simulink library "halout"  (R2021b)
settings: Solver=VariableStepAuto  StartTime=0.0  StopTime=10.0  RelTol=1e-3
undefined symbols (not defined in the file): C_TASK_5MS_S, FALSE, KHAL_CAN1FD1APS3E2E_flg, KHAL_CAN1FD1APS3TxReq_flg, KHAL_CAN1FD1VCU2E2E_flg, KHAL_CAN1FD1VCU2TxReq_flg, KHAL_CAN1FD1VCU3E2E_flg, KHAL_CAN1FD1VCU3TxReq_flg, KHAL_CAN1TxReq_flg, KHAL_CAN1VMCFCM1E2E_flg, KHAL_CAN1VMCFCM1TxReq_flg, KHAL_CAN2TxReq_flg, KHAL_CAN3FD3VCU1toNIDECTxReq_flg, KHAL_CAN3FD3VCU1TxReq_flg, KHAL_CAN3FD3VCU2E2E_flg, KHAL_CAN3FD3VCU2toNIDECE2E_flg, KHAL_CAN3FD3VCU2toNIDECTxReq_flg, KHAL_CAN3FD3VCU2TxReq_flg, KHAL_CAN3TxReq_flg, KHAL_CAN4FD4CE1000E2E_flg, KHAL_CAN4FD4CE1000TxReq_flg, KHAL_CAN4TxReq_flg, KHAL_CAN5TxReq_flg, KHAL_CAN6FD6APS3E2E_flg, KHAL_CAN6FD6APS3TxReq_flg, KHAL_CAN6FD6VCU2E2E_flg, KHAL_CAN6FD6VCU2TxReq_flg, KHAL_CAN6TxReq_flg, ONE_INT, TRUE, ZERO_INT
libraries: FVT_lib x549, simulink x244
(part 16 of 27)

== system halout/HAL_OUT/CAN1/FD1_VCU2_0x154/Byte_3 ==
  Fr_DriverTq : Inport
  BitwiseOR : simulink/Logic and Bit Operations/Bitwise Operator  logicop=OR  UseBitMask=off  BitMask=bin2dec('11011001')  BitMaskRealWorld=Stored Integer
  SignalPack : FVT_lib/hal/SignalPack  RightShiftCnt=0  BitMask=2^8-1  LeftShiftCnt=0
  UnitConverter : DataTypeConversion  OutDataTypeStr=uint8  RndMeth=Round
  UnitConverter1 : DataTypeConversion  OutDataTypeStr=uint16  RndMeth=Round
  convert_out : FVT_lib/hal/convert_out  gain=0.5  offset=-5300
  Byte_3 : Outport
  wires:
  BitwiseOR/1 -> Byte_3/1
  UnitConverter/1 -> BitwiseOR/1
  SignalPack/1 -> UnitConverter/1
  UnitConverter1/1 -> SignalPack/1
  convert_out/1 -> UnitConverter1/1
  Fr_DriverTq/1 -> convert_out/1

== system halout/HAL_OUT/CAN1/FD1_VCU2_0x154/Byte_4 ==
  Rr_DriverTq : Inport
  BitwiseOR : simulink/Logic and Bit Operations/Bitwise Operator  logicop=OR  UseBitMask=off  BitMask=bin2dec('11011001')  BitMaskRealWorld=Stored Integer
  SignalPack : FVT_lib/hal/SignalPack  RightShiftCnt=8  BitMask=2^8-1  LeftShiftCnt=0
  UnitConverter : DataTypeConversion  OutDataTypeStr=uint8  RndMeth=Round
  UnitConverter1 : DataTypeConversion  OutDataTypeStr=uint16  RndMeth=Round
  convert_out : FVT_lib/hal/convert_out  gain=0.5  offset=-5300
  Byte_4 : Outport
  wires:
  BitwiseOR/1 -> Byte_4/1
  UnitConverter/1 -> BitwiseOR/1
  SignalPack/1 -> UnitConverter/1
  UnitConverter1/1 -> SignalPack/1
  convert_out/1 -> UnitConverter1/1
  Rr_DriverTq/1 -> convert_out/1

== system halout/HAL_OUT/CAN1/FD1_VCU2_0x154/Byte_5 ==
  Rr_DriverTq : Inport
  BitwiseOR : simulink/Logic and Bit Operations/Bitwise Operator  logicop=OR  UseBitMask=off  BitMask=bin2dec('11011001')  BitMaskRealWorld=Stored Integer
  SignalPack : FVT_lib/hal/SignalPack  RightShiftCnt=0  BitMask=2^8-1  LeftShiftCnt=0
  UnitConverter : DataTypeConversion  OutDataTypeStr=uint8  RndMeth=Round
  UnitConverter1 : DataTypeConversion  OutDataTypeStr=uint16  RndMeth=Round
  convert_out : FVT_lib/hal/convert_out  gain=0.5  offset=-5300
  Byte_5 : Outport
  wires:
  BitwiseOR/1 -> Byte_5/1
  UnitConverter/1 -> BitwiseOR/1
  SignalPack/1 -> UnitConverter/1
  UnitConverter1/1 -> SignalPack/1
  convert_out/1 -> UnitConverter1/1
  Rr_DriverTq/1 -> convert_out/1

== system halout/HAL_OUT/CAN1/FD1_VCU2_0x154/Byte_6 ==
  ACC_CtrlAvail : Inport
  AccPedal_Override : Inport  Port=2
  BitwiseOR : simulink/Logic and Bit Operations/Bitwise Operator  logicop=OR  UseBitMask=off  NumInputPorts=2  BitMask=bin2dec('11011001')  BitMaskRealWorld=Stored Integer
  SignalPack : FVT_lib/hal/SignalPack  RightShiftCnt=0  BitMask=2^1-1  LeftShiftCnt=7
  SignalPack1 : FVT_lib/hal/SignalPack  RightShiftCnt=0  BitMask=2^1-1  LeftShiftCnt=6
  UnitConverter{,1..3} (4 alike) : DataTypeConversion  OutDataTypeStr=uint8  RndMeth=Round
  Byte_6 : Outport
  wires:
  BitwiseOR/1 -> Byte_6/1
  UnitConverter/1 -> BitwiseOR/1
  SignalPack/1 -> UnitConverter/1
  UnitConverter1/1 -> SignalPack/1
  ACC_CtrlAvail/1 -> UnitConverter1/1
  UnitConverter2/1 -> BitwiseOR/2
  SignalPack1/1 -> UnitConverter2/1
  UnitConverter3/1 -> SignalPack1/1
  AccPedal_Override/1 -> UnitConverter3/1

== system halout/HAL_OUT/CAN1/FD1_VCU2_0x154/CRC8_IfAction_Tx ==
  CAN_E2E_flg : Inport
  DataID1 : Inport  Port=2
  DataID2 : Inport  Port=3
  RawData : Inport  Port=4
  Data Type Conversion : DataTypeConversion  OutDataTypeStr=uint8
  If : If
  If Action Subsystem : Subsystem  TreatAsAtomicUnit=on
  If Action Subsystem1 : Subsystem  TreatAsAtomicUnit=on
  Merge : Merge
  CRC8 : Outport
  wires:
  If/2 -> If Action Subsystem/Action
  If/1 -> If Action Subsystem1/Action
  CAN_E2E_flg/1 -> [CAN_E2E_flg]
  DataID1/1 -> [DataID1]
  DataID2/1 -> [DataID2]
  RawData/1 -> [RawData]
  [CAN_E2E_flg] -> Data Type Conversion/1
  [DataID1] -> If Action Subsystem1/1(CAN_E2E_ID1)
  [DataID2] -> If Action Subsystem1/2(CAN_E2E_ID2)
  [RawData] -> If Action Subsystem1/3(Byte1)
  [RawData] -> If Action Subsystem/1(Byte1)
  If Action Subsystem1/1(CRC8_E2EResult) -> Merge/1
  If Action Subsystem/1(CRC8_Result) -> Merge/2
  Merge/1 -> CRC8/1
  Data Type Conversion/1 -> If/1

== system halout/HAL_OUT/CAN1/FD1_VCU2_0x154/CSVCU2CAN1 ==
  CSVCU2CAN1 : Inport
  Data Type Conversion : DataTypeConversion  OutDataTypeStr=uint8  RndMeth=Round
  CAN1_CS_VCU2_CAN1 : Outport
  wires:
  Data Type Conversion/1 -> CAN1_CS_VCU2_CAN1/1
  CSVCU2CAN1/1 -> Data Type Conversion/1

== system halout/HAL_OUT/CAN1/FD1_VCU2_0x154/DriverTq ==
  DriverTq : Inport
  Data Type Conversion : DataTypeConversion  OutDataTypeStr=uint16  RndMeth=Round
  convert_out : FVT_lib/hal/convert_out  gain=1  offset=-4300
  CAN1_DriverTq : Outport
  wires:
  Data Type Conversion/1 -> CAN1_DriverTq/1
  convert_out/1 -> Data Type Conversion/1
  DriverTq/1 -> convert_out/1

== system halout/HAL_OUT/CAN1/FD1_VCU2_0x154/FrDriverTq ==
  FrDriverTq : Inport
  Data Type Conversion : DataTypeConversion  OutDataTypeStr=uint16  RndMeth=Round
  convert_out : FVT_lib/hal/convert_out  gain=0.5  offset=-5300
  CAN1_Fr_DriverTq : Outport
  wires:
  Data Type Conversion/1 -> CAN1_Fr_DriverTq/1
  convert_out/1 -> Data Type Conversion/1
  FrDriverTq/1 -> convert_out/1

== system halout/HAL_OUT/CAN1/FD1_VCU2_0x154/RCVCU2CAN1 ==
  RCVCU2CAN1 : Inport
  Data Type Conversion : DataTypeConversion  OutDataTypeStr=uint8  RndMeth=Round
  CAN1_RC_VCU2_CAN1 : Outport
  wires:
  Data Type Conversion/1 -> CAN1_RC_VCU2_CAN1/1
  RCVCU2CAN1/1 -> Data Type Conversion/1

== system halout/HAL_OUT/CAN1/FD1_VCU2_0x154/RrDriverTq ==
  RrDriverTq : Inport
  Data Type Conversion : DataTypeConversion  OutDataTypeStr=uint16  RndMeth=Round
  convert_out : FVT_lib/hal/convert_out  gain=0.5  offset=-5300
  CAN1_Rr_DriverTq : Outport
  wires:
  Data Type Conversion/1 -> CAN1_Rr_DriverTq/1
  convert_out/1 -> Data Type Conversion/1
  RrDriverTq/1 -> convert_out/1

== system halout/HAL_OUT/CAN1/FD1_VCU2_0x154/VehActPwr ==
  VehActPwr : Inport
  Data Type Conversion : DataTypeConversion  OutDataTypeStr=uint32  RndMeth=Round
  convert_out : FVT_lib/hal/convert_out  gain=1  offset=-600000
  CAN1_VehActPwr : Outport
  wires:
  Data Type Conversion/1 -> CAN1_VehActPwr/1
  convert_out/1 -> Data Type Conversion/1
  VehActPwr/1 -> convert_out/1

== system halout/HAL_OUT/CAN1/FD1_VCU3_0x159/Byte_0 ==
  CS_VCU3_CAN1 : Inport
  BitwiseOR : simulink/Logic and Bit Operations/Bitwise Operator  logicop=OR  UseBitMask=off  BitMask=bin2dec('11011001')  BitMaskRealWorld=Stored Integer
  SignalPack : FVT_lib/hal/SignalPack  RightShiftCnt=0  BitMask=2^8-1  LeftShiftCnt=0
  UnitConverter : DataTypeConversion  OutDataTypeStr=uint8  RndMeth=Round
  UnitConverter1 : DataTypeConversion  OutDataTypeStr=uint8  RndMeth=Round
  Byte_0 : Outport
  wires:
  BitwiseOR/1 -> Byte_0/1
  UnitConverter/1 -> BitwiseOR/1
  SignalPack/1 -> UnitConverter/1
  UnitConverter1/1 -> SignalPack/1
  CS_VCU3_CAN1/1 -> UnitConverter1/1

== system halout/HAL_OUT/CAN1/FD1_VCU3_0x159/Byte_1 ==
  RC_VCU3_CAN1 : Inport
  BitwiseOR : simulink/Logic and Bit Operations/Bitwise Operator  logicop=OR  UseBitMask=off  BitMask=bin2dec('11011001')  BitMaskRealWorld=Stored Integer
  SignalPack : FVT_lib/hal/SignalPack  RightShiftCnt=0  BitMask=2^4-1  LeftShiftCnt=0
  UnitConverter : DataTypeConversion  OutDataTypeStr=uint8  RndMeth=Round
  UnitConverter1 : DataTypeConversion  OutDataTypeStr=uint8  RndMeth=Round
  Byte_1 : Outport
  wires:
  BitwiseOR/1 -> Byte_1/1
  UnitConverter/1 -> BitwiseOR/1
  SignalPack/1 -> UnitConverter/1
  UnitConverter1/1 -> SignalPack/1
  RC_VCU3_CAN1/1 -> UnitConverter1/1

== system halout/HAL_OUT/CAN1/FD1_VCU3_0x159/Byte_10 ==
  Rr_EDURealDrvOrBRgnTq : Inport
  BitwiseOR : simulink/Logic and Bit Operations/Bitwise Operator  logicop=OR  UseBitMask=off  BitMask=bin2dec('11011001')  BitMaskRealWorld=Stored Integer
  SignalPack : FVT_lib/hal/SignalPack  RightShiftCnt=8  BitMask=2^8-1  LeftShiftCnt=0
  UnitConverter : DataTypeConversion  OutDataTypeStr=uint8  RndMeth=Round
  UnitConverter1 : DataTypeConversion  OutDataTypeStr=uint16  RndMeth=Round
  convert_out : FVT_lib/hal/convert_out  gain=0.5  offset=-5300
  Byte_10 : Outport
  wires:
  BitwiseOR/1 -> Byte_10/1
  UnitConverter/1 -> BitwiseOR/1
  SignalPack/1 -> UnitConverter/1
  UnitConverter1/1 -> SignalPack/1
  convert_out/1 -> UnitConverter1/1
  Rr_EDURealDrvOrBRgnTq/1 -> convert_out/1

== system halout/HAL_OUT/CAN1/FD1_VCU3_0x159/Byte_11 ==
  Rr_EDURealDrvOrBRgnTq : Inport
  BitwiseOR : simulink/Logic and Bit Operations/Bitwise Operator  logicop=OR  UseBitMask=off  BitMask=bin2dec('11011001')  BitMaskRealWorld=Stored Integer
  SignalPack : FVT_lib/hal/SignalPack  RightShiftCnt=0  BitMask=2^8-1  LeftShiftCnt=0
  UnitConverter : DataTypeConversion  OutDataTypeStr=uint8  RndMeth=Round
  UnitConverter1 : DataTypeConversion  OutDataTypeStr=uint16  RndMeth=Round
  convert_out : FVT_lib/hal/convert_out  gain=0.5  offset=-5300
  Byte_11 : Outport
  wires:
  BitwiseOR/1 -> Byte_11/1
  UnitConverter/1 -> BitwiseOR/1
  SignalPack/1 -> UnitConverter/1
  UnitConverter1/1 -> SignalPack/1
  convert_out/1 -> UnitConverter1/1
  Rr_EDURealDrvOrBRgnTq/1 -> convert_out/1

== system halout/HAL_OUT/CAN1/FD1_VCU3_0x159/Byte_12 ==
  Fr_EDUAvailBrkRgnTqValid : Inport
  Fr_EDUSpd : Inport  Port=2
  Rr_EDUAvailBrkRgnTqValid : Inport  Port=3
  BitwiseOR : simulink/Logic and Bit Operations/Bitwise Operator  logicop=OR  UseBitMask=off  NumInputPorts=3  BitMask=bin2dec('11011001')  BitMaskRealWorld=Stored Integer
  SignalPack : FVT_lib/hal/SignalPack  RightShiftCnt=0  BitMask=2^1-1  LeftShiftCnt=6
  SignalPack1 : FVT_lib/hal/SignalPack  RightShiftCnt=8  BitMask=2^4-1  LeftShiftCnt=0
  SignalPack2 : FVT_lib/hal/SignalPack  RightShiftCnt=0  BitMask=2^1-1  LeftShiftCnt=7
  UnitConverter{,1..2,4..5} (5 alike) : DataTypeConversion  OutDataTypeStr=uint8  RndMeth=Round
  UnitConverter3 : DataTypeConversion  OutDataTypeStr=uint16  RndMeth=Round
  convert_out : FVT_lib/hal/convert_out  gain=1  offset=-2000
  Byte_12 : Outport
  wires:
  BitwiseOR/1 -> Byte_12/1
  UnitConverter/1 -> BitwiseOR/1
  SignalPack/1 -> UnitConverter/1
  UnitConverter1/1 -> SignalPack/1
  Fr_EDUAvailBrkRgnTqValid/1 -> UnitConverter1/1
  UnitConverter2/1 -> BitwiseOR/2
  SignalPack1/1 -> UnitConverter2/1
  UnitConverter3/1 -> SignalPack1/1
  convert_out/1 -> UnitConverter3/1
  Fr_EDUSpd/1 -> convert_out/1
  UnitConverter4/1 -> BitwiseOR/3
  SignalPack2/1 -> UnitConverter4/1
  UnitConverter5/1 -> SignalPack2/1
  Rr_EDUAvailBrkRgnTqValid/1 -> UnitConverter5/1

== system halout/HAL_OUT/CAN1/FD1_VCU3_0x159/Byte_13 ==
  Fr_EDUSpd : Inport
  BitwiseOR : simulink/Logic and Bit Operations/Bitwise Operator  logicop=OR  UseBitMask=off  BitMask=bin2dec('11011001')  BitMaskRealWorld=Stored Integer
  SignalPack : FVT_lib/hal/SignalPack  RightShiftCnt=0  BitMask=2^8-1  LeftShiftCnt=0
  UnitConverter : DataTypeConversion  OutDataTypeStr=uint8  RndMeth=Round
  UnitConverter1 : DataTypeConversion  OutDataTypeStr=uint16  RndMeth=Round
  convert_out : FVT_lib/hal/convert_out  gain=1  offset=-2000
  Byte_13 : Outport
  wires:
  BitwiseOR/1 -> Byte_13/1
  UnitConverter/1 -> BitwiseOR/1
  SignalPack/1 -> UnitConverter/1
  UnitConverter1/1 -> SignalPack/1
  convert_out/1 -> UnitConverter1/1
  Fr_EDUSpd/1 -> convert_out/1

== system halout/HAL_OUT/CAN1/FD1_VCU3_0x159/Byte_14 ==
  Fr_EDURealARgnTq : Inport
  BitwiseOR : simulink/Logic and Bit Operations/Bitwise Operator  logicop=OR  UseBitMask=off  BitMask=bin2dec('11011001')  BitMaskRealWorld=Stored Integer
  SignalPack : FVT_lib/hal/SignalPack  RightShiftCnt=8  BitMask=2^8-1  LeftShiftCnt=0
  UnitConverter : DataTypeConversion  OutDataTypeStr=uint8  RndMeth=Round
  UnitConverter1 : DataTypeConversion  OutDataTypeStr=uint16  RndMeth=Round
  convert_out : FVT_lib/hal/convert_out  gain=1  offset=-5300
  Byte_14 : Outport
  wires:
  BitwiseOR/1 -> Byte_14/1
  UnitConverter/1 -> BitwiseOR/1
  SignalPack/1 -> UnitConverter/1
  UnitConverter1/1 -> SignalPack/1
  convert_out/1 -> UnitConverter1/1
  Fr_EDURealARgnTq/1 -> convert_out/1

== system halout/HAL_OUT/CAN1/FD1_VCU3_0x159/Byte_15 ==
  Fr_EDURealARgnTq : Inport
  BitwiseOR : simulink/Logic and Bit Operations/Bitwise Operator  logicop=OR  UseBitMask=off  BitMask=bin2dec('11011001')  BitMaskRealWorld=Stored Integer
  SignalPack : FVT_lib/hal/SignalPack  RightShiftCnt=0  BitMask=2^8-1  LeftShiftCnt=0
  UnitConverter : DataTypeConversion  OutDataTypeStr=uint8  RndMeth=Round
  UnitConverter1 : DataTypeConversion  OutDataTypeStr=uint16  RndMeth=Round
  convert_out : FVT_lib/hal/convert_out  gain=1  offset=-5300
  Byte_15 : Outport
  wires:
  BitwiseOR/1 -> Byte_15/1
  UnitConverter/1 -> BitwiseOR/1
  SignalPack/1 -> UnitConverter/1
  UnitConverter1/1 -> SignalPack/1
  convert_out/1 -> UnitConverter1/1
  Fr_EDURealARgnTq/1 -> convert_out/1

== system halout/HAL_OUT/CAN1/FD1_VCU3_0x159/Byte_16 ==
  Fr_EDUAvailBrkRgnTq : Inport
  BitwiseOR : simulink/Logic and Bit Operations/Bitwise Operator  logicop=OR  UseBitMask=off  BitMask=bin2dec('11011001')  BitMaskRealWorld=Stored Integer
  SignalPack : FVT_lib/hal/SignalPack  RightShiftCnt=8  BitMask=2^8-1  LeftShiftCnt=0
  UnitConverter : DataTypeConversion  OutDataTypeStr=uint8  RndMeth=Round
  UnitConverter1 : DataTypeConversion  OutDataTypeStr=uint16  RndMeth=Round
  convert_out : FVT_lib/hal/convert_out  gain=0.5  offset=-5300
  Byte_16 : Outport
  wires:
  BitwiseOR/1 -> Byte_16/1
  UnitConverter/1 -> BitwiseOR/1
  SignalPack/1 -> UnitConverter/1
  UnitConverter1/1 -> SignalPack/1
  convert_out/1 -> UnitConverter1/1
  Fr_EDUAvailBrkRgnTq/1 -> convert_out/1

== system halout/HAL_OUT/CAN1/FD1_VCU3_0x159/Byte_17 ==
  Fr_EDUAvailBrkRgnTq : Inport
  BitwiseOR : simulink/Logic and Bit Operations/Bitwise Operator  logicop=OR  UseBitMask=off  BitMask=bin2dec('11011001')  BitMaskRealWorld=Stored Integer
  SignalPack : FVT_lib/hal/SignalPack  RightShiftCnt=0  BitMask=2^8-1  LeftShiftCnt=0
  UnitConverter : DataTypeConversion  OutDataTypeStr=uint8  RndMeth=Round
  UnitConverter1 : DataTypeConversion  OutDataTypeStr=uint16  RndMeth=Round
  convert_out : FVT_lib/hal/convert_out  gain=0.5  offset=-5300
  Byte_17 : Outport
  wires:
  BitwiseOR/1 -> Byte_17/1
  UnitConverter/1 -> BitwiseOR/1
  SignalPack/1 -> UnitConverter/1
  UnitConverter1/1 -> SignalPack/1
  convert_out/1 -> UnitConverter1/1
  Fr_EDUAvailBrkRgnTq/1 -> convert_out/1

== system halout/HAL_OUT/CAN1/FD1_VCU3_0x159/Byte_18 ==
  Fr_EDURealDrvOrBRgnTq : Inport
  BitwiseOR : simulink/Logic and Bit Operations/Bitwise Operator  logicop=OR  UseBitMask=off  BitMask=bin2dec('11011001')  BitMaskRealWorld=Stored Integer
  SignalPack : FVT_lib/hal/SignalPack  RightShiftCnt=8  BitMask=2^8-1  LeftShiftCnt=0
  UnitConverter : DataTypeConversion  OutDataTypeStr=uint8  RndMeth=Round
  UnitConverter1 : DataTypeConversion  OutDataTypeStr=uint16  RndMeth=Round
  convert_out : FVT_lib/hal/convert_out  gain=0.5  offset=-5300
  Byte_18 : Outport
  wires:
  BitwiseOR/1 -> Byte_18/1
  UnitConverter/1 -> BitwiseOR/1
  SignalPack/1 -> UnitConverter/1
  UnitConverter1/1 -> SignalPack/1
  convert_out/1 -> UnitConverter1/1
  Fr_EDURealDrvOrBRgnTq/1 -> convert_out/1

== system halout/HAL_OUT/CAN1/FD1_VCU3_0x159/Byte_19 ==
  Fr_EDURealDrvOrBRgnTq : Inport
  BitwiseOR : simulink/Logic and Bit Operations/Bitwise Operator  logicop=OR  UseBitMask=off  BitMask=bin2dec('11011001')  BitMaskRealWorld=Stored Integer
  SignalPack : FVT_lib/hal/SignalPack  RightShiftCnt=0  BitMask=2^8-1  LeftShiftCnt=0
  UnitConverter : DataTypeConversion  OutDataTypeStr=uint8  RndMeth=Round
  UnitConverter1 : DataTypeConversion  OutDataTypeStr=uint16  RndMeth=Round
  convert_out : FVT_lib/hal/convert_out  gain=0.5  offset=-5300
  Byte_19 : Outport
  wires:
  BitwiseOR/1 -> Byte_19/1
  UnitConverter/1 -> BitwiseOR/1
  SignalPack/1 -> UnitConverter/1
  UnitConverter1/1 -> SignalPack/1
  convert_out/1 -> UnitConverter1/1
  Fr_EDURealDrvOrBRgnTq/1 -> convert_out/1

== system halout/HAL_OUT/CAN1/FD1_VCU3_0x159/Byte_3 ==
  Fr_EDUSpdValid : Inport
  Fr_RgnDecrSta : Inport  Port=2
  Fr_RgnPermSta : Inport  Port=3
  RgnAbnorSta : Inport  Port=4
  Rr_EDUSpdValid : Inport  Port=5
  Rr_RgnDecrSta : Inport  Port=6
  Rr_RgnPermSta : Inport  Port=7
  BitwiseOR : simulink/Logic and Bit Operations/Bitwise Operator  logicop=OR  UseBitMask=off  NumInputPorts=7  BitMask=bin2dec('11011001')  BitMaskRealWorld=Stored Integer
  SignalPack : FVT_lib/hal/SignalPack  RightShiftCnt=0  BitMask=2^1-1  LeftShiftCnt=6
  SignalPack1 : FVT_lib/hal/SignalPack  RightShiftCnt=0  BitMask=2^1-1  LeftShiftCnt=3
  SignalPack2 : FVT_lib/hal/SignalPack  RightShiftCnt=0  BitMask=2^1-1  LeftShiftCnt=1
  SignalPack3 : FVT_lib/hal/SignalPack  RightShiftCnt=0  BitMask=2^1-1  LeftShiftCnt=4
  SignalPack4 : FVT_lib/hal/SignalPack  RightShiftCnt=0  BitMask=2^1-1  LeftShiftCnt=5
  SignalPack5 : FVT_lib/hal/SignalPack  RightShiftCnt=0  BitMask=2^1-1  LeftShiftCnt=2
  SignalPack6 : FVT_lib/hal/SignalPack  RightShiftCnt=0  BitMask=2^1-1  LeftShiftCnt=0
  UnitConverter{,1..13} (14 alike) : DataTypeConversion  OutDataTypeStr=uint8  RndMeth=Round
  Byte_3 : Outport
  wires:
  BitwiseOR/1 -> Byte_3/1
  UnitConverter/1 -> BitwiseOR/1
  SignalPack/1 -> UnitConverter/1
  UnitConverter1/1 -> SignalPack/1
  Fr_EDUSpdValid/1 -> UnitConverter1/1
  UnitConverter2/1 -> BitwiseOR/2
  SignalPack1/1 -> UnitConverter2/1
  UnitConverter3/1 -> SignalPack1/1
  Fr_RgnDecrSta/1 -> UnitConverter3/1
  UnitConverter4/1 -> BitwiseOR/3
  SignalPack2/1 -> UnitConverter4/1
  UnitConverter5/1 -> SignalPack2/1
  Fr_RgnPermSta/1 -> UnitConverter5/1
  UnitConverter6/1 -> BitwiseOR/4
  SignalPack3/1 -> UnitConverter6/1
  UnitConverter7/1 -> SignalPack3/1
  RgnAbnorSta/1 -> UnitConverter7/1
  UnitConverter8/1 -> BitwiseOR/5
  SignalPack4/1 -> UnitConverter8/1
  UnitConverter9/1 -> SignalPack4/1
  Rr_EDUSpdValid/1 -> UnitConverter9/1
  UnitConverter10/1 -> BitwiseOR/6
  SignalPack5/1 -> UnitConverter10/1
  UnitConverter11/1 -> SignalPack5/1
  Rr_RgnDecrSta/1 -> UnitConverter11/1
  UnitConverter12/1 -> BitwiseOR/7
  SignalPack6/1 -> UnitConverter12/1
  UnitConverter13/1 -> SignalPack6/1
  Rr_RgnPermSta/1 -> UnitConverter13/1

== system halout/HAL_OUT/CAN1/FD1_VCU3_0x159/Byte_4 ==
  EquivAccPedalSWSta : Inport
  PTCS_PermSta : Inport  Port=2
  Rr_EDUSpd : Inport  Port=3
  BitwiseOR : simulink/Logic and Bit Operations/Bitwise Operator  logicop=OR  UseBitMask=off  NumInputPorts=3  BitMask=bin2dec('11011001')  BitMaskRealWorld=Stored Integer
  SignalPack : FVT_lib/hal/SignalPack  RightShiftCnt=0  BitMask=2^1-1  LeftShiftCnt=6
  SignalPack1 : FVT_lib/hal/SignalPack  RightShiftCnt=0  BitMask=2^1-1  LeftShiftCnt=7
  SignalPack2 : FVT_lib/hal/SignalPack  RightShiftCnt=8  BitMask=2^4-1  LeftShiftCnt=0
  UnitConverter{,1..4} (5 alike) : DataTypeConversion  OutDataTypeStr=uint8  RndMeth=Round
  UnitConverter5 : DataTypeConversion  OutDataTypeStr=uint16  RndMeth=Round
  convert_out : FVT_lib/hal/convert_out  gain=1  offset=-2000
  Byte_4 : Outport
  wires:
  BitwiseOR/1 -> Byte_4/1
  UnitConverter/1 -> BitwiseOR/1
  SignalPack/1 -> UnitConverter/1
  UnitConverter1/1 -> SignalPack/1
  EquivAccPedalSWSta/1 -> UnitConverter1/1
  UnitConverter2/1 -> BitwiseOR/2
  SignalPack1/1 -> UnitConverter2/1
  UnitConverter3/1 -> SignalPack1/1
  PTCS_PermSta/1 -> UnitConverter3/1
  UnitConverter4/1 -> BitwiseOR/3
  SignalPack2/1 -> UnitConverter4/1
  UnitConverter5/1 -> SignalPack2/1
  convert_out/1 -> UnitConverter5/1
  Rr_EDUSpd/1 -> convert_out/1

== system halout/HAL_OUT/CAN1/FD1_VCU3_0x159/Byte_5 ==
  Rr_EDUSpd : Inport
  BitwiseOR : simulink/Logic and Bit Operations/Bitwise Operator  logicop=OR  UseBitMask=off  BitMask=bin2dec('11011001')  BitMaskRealWorld=Stored Integer
  SignalPack : FVT_lib/hal/SignalPack  RightShiftCnt=0  BitMask=2^8-1  LeftShiftCnt=0
  UnitConverter : DataTypeConversion  OutDataTypeStr=uint8  RndMeth=Round
  UnitConverter1 : DataTypeConversion  OutDataTypeStr=uint16  RndMeth=Round
  convert_out : FVT_lib/hal/convert_out  gain=1  offset=-2000
  Byte_5 : Outport
  wires:
  BitwiseOR/1 -> Byte_5/1
  UnitConverter/1 -> BitwiseOR/1
  SignalPack/1 -> UnitConverter/1
  UnitConverter1/1 -> SignalPack/1
  convert_out/1 -> UnitConverter1/1
  Rr_EDUSpd/1 -> convert_out/1

== system halout/HAL_OUT/CAN1/FD1_VCU3_0x159/Byte_6 ==
  Rr_EDURealARgnTq : Inport
  BitwiseOR : simulink/Logic and Bit Operations/Bitwise Operator  logicop=OR  UseBitMask=off  BitMask=bin2dec('11011001')  BitMaskRealWorld=Stored Integer
  SignalPack : FVT_lib/hal/SignalPack  RightShiftCnt=8  BitMask=2^8-1  LeftShiftCnt=0
  UnitConverter : DataTypeConversion  OutDataTypeStr=uint8  RndMeth=Round
  UnitConverter1 : DataTypeConversion  OutDataTypeStr=uint16  RndMeth=Round
  convert_out : FVT_lib/hal/convert_out  gain=1  offset=-5300
  Byte_6 : Outport
  wires:
  BitwiseOR/1 -> Byte_6/1
  UnitConverter/1 -> BitwiseOR/1
  SignalPack/1 -> UnitConverter/1
  UnitConverter1/1 -> SignalPack/1
  convert_out/1 -> UnitConverter1/1
  Rr_EDURealARgnTq/1 -> convert_out/1

== system halout/HAL_OUT/CAN1/FD1_VCU3_0x159/Byte_7 ==
  Rr_EDURealARgnTq : Inport
  BitwiseOR : simulink/Logic and Bit Operations/Bitwise Operator  logicop=OR  UseBitMask=off  BitMask=bin2dec('11011001')  BitMaskRealWorld=Stored Integer
  SignalPack : FVT_lib/hal/SignalPack  RightShiftCnt=0  BitMask=2^8-1  LeftShiftCnt=0
  UnitConverter : DataTypeConversion  OutDataTypeStr=uint8  RndMeth=Round
  UnitConverter1 : DataTypeConversion  OutDataTypeStr=uint16  RndMeth=Round
  convert_out : FVT_lib/hal/convert_out  gain=1  offset=-5300
  Byte_7 : Outport
  wires:
  BitwiseOR/1 -> Byte_7/1
  UnitConverter/1 -> BitwiseOR/1
  SignalPack/1 -> UnitConverter/1
  UnitConverter1/1 -> SignalPack/1
  convert_out/1 -> UnitConverter1/1
  Rr_EDURealARgnTq/1 -> convert_out/1

== system halout/HAL_OUT/CAN1/FD1_VCU3_0x159/Byte_8 ==
  Rr_EDUAvailBrkRgnTq : Inport
  BitwiseOR : simulink/Logic and Bit Operations/Bitwise Operator  logicop=OR  UseBitMask=off  BitMask=bin2dec('11011001')  BitMaskRealWorld=Stored Integer
  SignalPack : FVT_lib/hal/SignalPack  RightShiftCnt=8  BitMask=2^8-1  LeftShiftCnt=0
  UnitConverter : DataTypeConversion  OutDataTypeStr=uint8  RndMeth=Round
  UnitConverter1 : DataTypeConversion  OutDataTypeStr=uint16  RndMeth=Round
  convert_out : FVT_lib/hal/convert_out  gain=0.5  offset=-5300
  Byte_8 : Outport
  wires:
  BitwiseOR/1 -> Byte_8/1
  UnitConverter/1 -> BitwiseOR/1
  SignalPack/1 -> UnitConverter/1
  UnitConverter1/1 -> SignalPack/1
  convert_out/1 -> UnitConverter1/1
  Rr_EDUAvailBrkRgnTq/1 -> convert_out/1

== system halout/HAL_OUT/CAN1/FD1_VCU3_0x159/Byte_9 ==
  Rr_EDUAvailBrkRgnTq : Inport
  BitwiseOR : simulink/Logic and Bit Operations/Bitwise Operator  logicop=OR  UseBitMask=off  BitMask=bin2dec('11011001')  BitMaskRealWorld=Stored Integer
  SignalPack : FVT_lib/hal/SignalPack  RightShiftCnt=0  BitMask=2^8-1  LeftShiftCnt=0
  UnitConverter : DataTypeConversion  OutDataTypeStr=uint8  RndMeth=Round
  UnitConverter1 : DataTypeConversion  OutDataTypeStr=uint16  RndMeth=Round
  convert_out : FVT_lib/hal/convert_out  gain=0.5  offset=-5300
  Byte_9 : Outport
  wires:
  BitwiseOR/1 -> Byte_9/1
  UnitConverter/1 -> BitwiseOR/1
  SignalPack/1 -> UnitConverter/1
  UnitConverter1/1 -> SignalPack/1
  convert_out/1 -> UnitConverter1/1
  Rr_EDUAvailBrkRgnTq/1 -> convert_out/1

== system halout/HAL_OUT/CAN1/FD1_VCU3_0x159/CRC8_IfAction_Tx ==
  CAN_E2E_flg : Inport
  DataID1 : Inport  Port=2
  DataID2 : Inport  Port=3
  RawData : Inport  Port=4
  Data Type Conversion : DataTypeConversion  OutDataTypeStr=uint8
  If : If
  If Action Subsystem : Subsystem  TreatAsAtomicUnit=on
  If Action Subsystem1 : Subsystem  TreatAsAtomicUnit=on
  Merge : Merge
  CRC8 : Outport
  wires:
  If/2 -> If Action Subsystem/Action
  If/1 -> If Action Subsystem1/Action
  CAN_E2E_flg/1 -> [CAN_E2E_flg]
  DataID1/1 -> [DataID1]
  DataID2/1 -> [DataID2]
  RawData/1 -> [RawData]
  [CAN_E2E_flg] -> Data Type Conversion/1
  [DataID1] -> If Action Subsystem1/1(CAN_E2E_ID1)
  [DataID2] -> If Action Subsystem1/2(CAN_E2E_ID2)
  [RawData] -> If Action Subsystem1/3(Byte1)
  [RawData] -> If Action Subsystem/1(Byte1)
  If Action Subsystem1/1(CRC8_E2EResult) -> Merge/1
  If Action Subsystem/1(CRC8_Result) -> Merge/2
  Merge/1 -> CRC8/1
  Data Type Conversion/1 -> If/1

== system halout/HAL_OUT/CAN1/FD1_VCU3_0x159/CSVCU3CAN1 ==
  CSVCU3CAN1 : Inport
  Data Type Conversion : DataTypeConversion  OutDataTypeStr=uint8  RndMeth=Round
  CAN1_CS_VCU3_CAN1 : Outport
  wires:
  Data Type Conversion/1 -> CAN1_CS_VCU3_CAN1/1
  CSVCU3CAN1/1 -> Data Type Conversion/1

== system halout/HAL_OUT/CAN1/FD1_VCU3_0x159/EquivAccPedalSWSta ==
  EquivAccPedalSWSta : Inport
  Data Type Conversion : DataTypeConversion  OutDataTypeStr=uint8  RndMeth=Round
  CAN1_EquivAccPedalSWSta : Outport
  wires:
  Data Type Conversion/1 -> CAN1_EquivAccPedalSWSta/1
  EquivAccPedalSWSta/1 -> Data Type Conversion/1

== system halout/HAL_OUT/CAN1/FD1_VCU3_0x159/FrEDUAvailBrkRgnTq ==
  FrEDUAvailBrkRgnTq : Inport
  Data Type Conversion : DataTypeConversion  OutDataTypeStr=uint16  RndMeth=Round
  convert_out : FVT_lib/hal/convert_out  gain=0.5  offset=-5300
  CAN1_Fr_EDUAvailBrkRgnTq : Outport
  wires:
  Data Type Conversion/1 -> CAN1_Fr_EDUAvailBrkRgnTq/1
  convert_out/1 -> Data Type Conversion/1
  FrEDUAvailBrkRgnTq/1 -> convert_out/1

== system halout/HAL_OUT/CAN1/FD1_VCU3_0x159/FrEDUAvailBrkRgnTqValid ==
  FrEDUAvailBrkRgnTqValid : Inport
  Data Type Conversion : DataTypeConversion  OutDataTypeStr=uint8  RndMeth=Round
  CAN1_Fr_EDUAvailBrkRgnTqValid : Outport
  wires:
  Data Type Conversion/1 -> CAN1_Fr_EDUAvailBrkRgnTqValid/1
  FrEDUAvailBrkRgnTqValid/1 -> Data Type Conversion/1

== system halout/HAL_OUT/CAN1/FD1_VCU3_0x159/FrEDURealARgnTq ==
  FrEDURealARgnTq : Inport
  Data Type Conversion : DataTypeConversion  OutDataTypeStr=uint16  RndMeth=Round
  convert_out : FVT_lib/hal/convert_out  gain=1  offset=-5300
  CAN1_Fr_EDURealARgnTq : Outport
  wires:
  Data Type Conversion/1 -> CAN1_Fr_EDURealARgnTq/1
  convert_out/1 -> Data Type Conversion/1
  FrEDURealARgnTq/1 -> convert_out/1

== system halout/HAL_OUT/CAN1/FD1_VCU3_0x159/FrEDURealDrvOrBRgnTq ==
  FrEDURealDrvOrBRgnTq : Inport
  Data Type Conversion : DataTypeConversion  OutDataTypeStr=uint16  RndMeth=Round
  convert_out : FVT_lib/hal/convert_out  gain=0.5  offset=-5300
  CAN1_Fr_EDURealDrvOrBRgnTq : Outport
  wires:
  Data Type Conversion/1 -> CAN1_Fr_EDURealDrvOrBRgnTq/1
  convert_out/1 -> Data Type Conversion/1
  FrEDURealDrvOrBRgnTq/1 -> convert_out/1

== system halout/HAL_OUT/CAN1/FD1_VCU3_0x159/FrEDUSpd ==
  FrEDUSpd : Inport
  Data Type Conversion : DataTypeConversion  OutDataTypeStr=uint16  RndMeth=Round
  convert_out : FVT_lib/hal/convert_out  gain=1  offset=-2000
  CAN1_Fr_EDUSpd : Outport
  wires:
  Data Type Conversion/1 -> CAN1_Fr_EDUSpd/1
  convert_out/1 -> Data Type Conversion/1
  FrEDUSpd/1 -> convert_out/1

== system halout/HAL_OUT/CAN1/FD1_VCU3_0x159/FrEDUSpdValid ==
  FrEDUSpdValid : Inport
  Data Type Conversion : DataTypeConversion  OutDataTypeStr=uint8  RndMeth=Round
  CAN1_Fr_EDUSpdValid : Outport
  wires:
  Data Type Conversion/1 -> CAN1_Fr_EDUSpdValid/1
  FrEDUSpdValid/1 -> Data Type Conversion/1

== system halout/HAL_OUT/CAN1/FD1_VCU3_0x159/FrRgnDecrSta ==
  FrRgnDecrSta : Inport
  Data Type Conversion : DataTypeConversion  OutDataTypeStr=uint8  RndMeth=Round
  CAN1_Fr_RgnDecrSta : Outport
  wires:
  Data Type Conversion/1 -> CAN1_Fr_RgnDecrSta/1
  FrRgnDecrSta/1 -> Data Type Conversion/1

== system halout/HAL_OUT/CAN1/FD1_VCU3_0x159/FrRgnPermSta ==
  FrRgnPermSta : Inport
  Data Type Conversion : DataTypeConversion  OutDataTypeStr=uint8  RndMeth=Round
  CAN1_Fr_RgnPermSta : Outport
  wires:
  Data Type Conversion/1 -> CAN1_Fr_RgnPermSta/1
  FrRgnPermSta/1 -> Data Type Conversion/1

== system halout/HAL_OUT/CAN1/FD1_VCU3_0x159/PTCSPermSta ==
  PTCSPermSta : Inport
  Data Type Conversion : DataTypeConversion  OutDataTypeStr=uint8  RndMeth=Round
  CAN1_PTCS_PermSta : Outport
  wires:
  Data Type Conversion/1 -> CAN1_PTCS_PermSta/1
  PTCSPermSta/1 -> Data Type Conversion/1

== system halout/HAL_OUT/CAN1/FD1_VCU3_0x159/RCVCU3CAN1 ==
  RCVCU3CAN1 : Inport
  Data Type Conversion : DataTypeConversion  OutDataTypeStr=uint8  RndMeth=Round
  CAN1_RC_VCU3_CAN1 : Outport
  wires:
  Data Type Conversion/1 -> CAN1_RC_VCU3_CAN1/1
  RCVCU3CAN1/1 -> Data Type Conversion/1

== system halout/HAL_OUT/CAN1/FD1_VCU3_0x159/RgnAbnorSta ==
  RgnAbnorSta : Inport
  Data Type Conversion : DataTypeConversion  OutDataTypeStr=uint8  RndMeth=Round
  CAN1_RgnAbnorSta : Outport
  wires:
  Data Type Conversion/1 -> CAN1_RgnAbnorSta/1
  RgnAbnorSta/1 -> Data Type Conversion/1

== system halout/HAL_OUT/CAN1/FD1_VCU3_0x159/RrEDUAvailBrkRgnTq ==
  RrEDUAvailBrkRgnTq : Inport
  Data Type Conversion : DataTypeConversion  OutDataTypeStr=uint16  RndMeth=Round
  convert_out : FVT_lib/hal/convert_out  gain=0.5  offset=-5300
  CAN1_Rr_EDUAvailBrkRgnTq : Outport
  wires:
  Data Type Conversion/1 -> CAN1_Rr_EDUAvailBrkRgnTq/1
  convert_out/1 -> Data Type Conversion/1
  RrEDUAvailBrkRgnTq/1 -> convert_out/1

== system halout/HAL_OUT/CAN1/FD1_VCU3_0x159/RrEDUAvailBrkRgnTqValid ==
  RrEDUAvailBrkRgnTqValid : Inport
  Data Type Conversion : DataTypeConversion  OutDataTypeStr=uint8  RndMeth=Round
  CAN1_Rr_EDUAvailBrkRgnTqValid : Outport
  wires:
  Data Type Conversion/1 -> CAN1_Rr_EDUAvailBrkRgnTqValid/1
  RrEDUAvailBrkRgnTqValid/1 -> Data Type Conversion/1

== system halout/HAL_OUT/CAN1/FD1_VCU3_0x159/RrEDURealARgnTq ==
  RrEDURealARgnTq : Inport
  Data Type Conversion : DataTypeConversion  OutDataTypeStr=uint16  RndMeth=Round
  convert_out : FVT_lib/hal/convert_out  gain=1  offset=-5300
  CAN1_Rr_EDURealARgnTq : Outport
  wires:
  Data Type Conversion/1 -> CAN1_Rr_EDURealARgnTq/1
  convert_out/1 -> Data Type Conversion/1
  RrEDURealARgnTq/1 -> convert_out/1

== system halout/HAL_OUT/CAN1/FD1_VCU3_0x159/RrEDURealDrvOrBRgnTq ==
  RrEDURealDrvOrBRgnTq : Inport
  Data Type Conversion : DataTypeConversion  OutDataTypeStr=uint16  RndMeth=Round
  convert_out : FVT_lib/hal/convert_out  gain=0.5  offset=-5300
  CAN1_Rr_EDURealDrvOrBRgnTq : Outport
  wires:
  Data Type Conversion/1 -> CAN1_Rr_EDURealDrvOrBRgnTq/1
  convert_out/1 -> Data Type Conversion/1
  RrEDURealDrvOrBRgnTq/1 -> convert_out/1

== system halout/HAL_OUT/CAN1/FD1_VCU3_0x159/RrEDUSpd ==
  RrEDUSpd : Inport
  Data Type Conversion : DataTypeConversion  OutDataTypeStr=uint16  RndMeth=Round
  convert_out : FVT_lib/hal/convert_out  gain=1  offset=-2000
  CAN1_Rr_EDUSpd : Outport
  wires:
  Data Type Conversion/1 -> CAN1_Rr_EDUSpd/1
  convert_out/1 -> Data Type Conversion/1
  RrEDUSpd/1 -> convert_out/1

== system halout/HAL_OUT/CAN1/FD1_VCU3_0x159/RrEDUSpdValid ==
  RrEDUSpdValid : Inport
  Data Type Conversion : DataTypeConversion  OutDataTypeStr=uint8  RndMeth=Round
  CAN1_Rr_EDUSpdValid : Outport
  wires:
  Data Type Conversion/1 -> CAN1_Rr_EDUSpdValid/1
  RrEDUSpdValid/1 -> Data Type Conversion/1

== system halout/HAL_OUT/CAN1/FD1_VCU3_0x159/RrRgnDecrSta ==
  RrRgnDecrSta : Inport
  Data Type Conversion : DataTypeConversion  OutDataTypeStr=uint8  RndMeth=Round
  CAN1_Rr_RgnDecrSta : Outport
  wires:
  Data Type Conversion/1 -> CAN1_Rr_RgnDecrSta/1
  RrRgnDecrSta/1 -> Data Type Conversion/1

== system halout/HAL_OUT/CAN1/FD1_VCU3_0x159/RrRgnPermSta ==
  RrRgnPermSta : Inport
  Data Type Conversion : DataTypeConversion  OutDataTypeStr=uint8  RndMeth=Round
  CAN1_Rr_RgnPermSta : Outport
  wires:
  Data Type Conversion/1 -> CAN1_Rr_RgnPermSta/1
  RrRgnPermSta/1 -> Data Type Conversion/1

== system halout/HAL_OUT/CAN1/FD1_VMC1_0x17F/AccCalcuPID ==
  AccCalcuPID : Inport
  Data Type Conversion : DataTypeConversion  OutDataTypeStr=uint16  RndMeth=Round
  convert_out : FVT_lib/hal/convert_out  gain=0.05  offset=-15
  CAN1_AccCalcuPID : Outport
  wires:
  Data Type Conversion/1 -> CAN1_AccCalcuPID/1
  convert_out/1 -> Data Type Conversion/1
  AccCalcuPID/1 -> convert_out/1

== system halout/HAL_OUT/CAN1/FD1_VMC1_0x17F/CCMSASpdWar ==
  CCMSASpdWar : Inport
  Data Type Conversion : DataTypeConversion  OutDataTypeStr=uint8  RndMeth=Round
  CAN1_CCMSA_SpdWar : Outport
  wires:
  Data Type Conversion/1 -> CAN1_CCMSA_SpdWar/1
  CCMSASpdWar/1 -> Data Type Conversion/1

== system halout/HAL_OUT/CAN1/FD1_VMC1_0x17F/DISCButtSta ==
  DISCButtSta : Inport
  Data Type Conversion : DataTypeConversion  OutDataTypeStr=uint8  RndMeth=Round
  CAN1_DISC_ButtSta : Outport
  wires:
  Data Type Conversion/1 -> CAN1_DISC_ButtSta/1
  DISCButtSta/1 -> Data Type Conversion/1

== system halout/HAL_OUT/CAN1/FD1_VMC1_0x17F/DISCDISCTargetSpd ==
  DISCDISCTargetSpd : Inport
  Data Type Conversion : DataTypeConversion  OutDataTypeStr=uint16  RndMeth=Round
  convert_out : FVT_lib/hal/convert_out  gain=0.125  offset=0
  CAN1_DISC_DISCTargetSpd : Outport
  wires:
  Data Type Conversion/1 -> CAN1_DISC_DISCTargetSpd/1
  convert_out/1 -> Data Type Conversion/1
  DISCDISCTargetSpd/1 -> convert_out/1

== system halout/HAL_OUT/CAN1/FD1_VMC1_0x17F/DISCDISCTurn ==
  DISCDISCTurn : Inport
  Data Type Conversion : DataTypeConversion  OutDataTypeStr=uint8  RndMeth=Round
  CAN1_DISC_DISCTurn : Outport
  wires:
  Data Type Conversion/1 -> CAN1_DISC_DISCTurn/1
  DISCDISCTurn/1 -> Data Type Conversion/1

== system halout/HAL_OUT/CAN1/FD1_VMC1_0x17F/DISCReqAcc ==
  DISCReqAcc : Inport
  Data Type Conversion : DataTypeConversion  OutDataTypeStr=uint16  RndMeth=Round
  convert_out : FVT_lib/hal/convert_out  gain=0.05  offset=-15
  CAN1_DISCReqAcc : Outport
  wires:
  Data Type Conversion/1 -> CAN1_DISCReqAcc/1
  convert_out/1 -> Data Type Conversion/1
  DISCReqAcc/1 -> convert_out/1

== system halout/HAL_OUT/CAN1/FD1_VMC1_0x17F/DISCSta ==
  DISCSta : Inport
  Data Type Conversion : DataTypeConversion  OutDataTypeStr=uint8  RndMeth=Round
  CAN1_DISC_Sta : Outport
  wires:
  Data Type Conversion/1 -> CAN1_DISC_Sta/1
  DISCSta/1 -> Data Type Conversion/1

== system halout/HAL_OUT/CAN1/FD1_VMC1_0x17F/FeatArbitrFinal ==
  FeatArbitrFinal : Inport
  Data Type Conversion : DataTypeConversion  OutDataTypeStr=uint8  RndMeth=Round
  CAN1_FeatArbitrFinal : Outport
  wires:
  Data Type Conversion/1 -> CAN1_FeatArbitrFinal/1
  FeatArbitrFinal/1 -> Data Type Conversion/1

== system halout/HAL_OUT/CAN1/FD1_VMC1_0x17F/FeatArbitrSta ==
  FeatArbitrSta : Inport
  Data Type Conversion : DataTypeConversion  OutDataTypeStr=uint8  RndMeth=Round
  CAN1_FeatArbitrSta : Outport
  wires:
  Data Type Conversion/1 -> CAN1_FeatArbitrSta/1
  FeatArbitrSta/1 -> Data Type Conversion/1

== system halout/HAL_OUT/CAN1/FD1_VMC1_0x17F/FeatReqSpd ==
  FeatReqSpd : Inport
  Data Type Conversion : DataTypeConversion  OutDataTypeStr=uint16  RndMeth=Round
  convert_out : FVT_lib/hal/convert_out  gain=0.125  offset=0
  CAN1_FeatReqSpd : Outport
  wires:
  Data Type Conversion/1 -> CAN1_FeatReqSpd/1
  convert_out/1 -> Data Type Conversion/1
  FeatReqSpd/1 -> convert_out/1

== system halout/HAL_OUT/CAN1/FD1_VMC1_0x17F/FeatSetSpdFinalraw32 ==
  FeatSetSpdFinalraw32 : Inport
  Data Type Conversion : DataTypeConversion  OutDataTypeStr=uint8  RndMeth=Round
  CAN1_FeatSetSpdFinal_raw32 : Outport
  wires:
  Data Type Conversion/1 -> CAN1_FeatSetSpdFinal_raw32/1
  FeatSetSpdFinalraw32/1 -> Data Type Conversion/1

== system halout/HAL_OUT/CAN1/FD1_VMC1_0x17F/FrontRearSlipRatioCtrl ==
  FrontRearSlipRatioCtrl : Inport
  Data Type Conversion : DataTypeConversion  OutDataTypeStr=uint8  RndMeth=Round
  CAN1_FrontRearSlipRatioCtrl : Outport
  wires:
  Data Type Conversion/1 -> CAN1_FrontRearSlipRatioCtrl/1
  FrontRearSlipRatioCtrl/1 -> Data Type Conversion/1

== system halout/HAL_OUT/CAN1/FD1_VMC1_0x17F/JerkPCT ==
  JerkPCT : Inport
  Data Type Conversion : DataTypeConversion  OutDataTypeStr=uint8  RndMeth=Round
  CAN1_JerkPCT : Outport
  wires:
  Data Type Conversion/1 -> CAN1_JerkPCT/1
  JerkPCT/1 -> Data Type Conversion/1

== system halout/HAL_OUT/CAN1/FD1_VMC1_0x17F/LatAccCtrl ==
  LatAccCtrl : Inport
  Data Type Conversion : DataTypeConversion  OutDataTypeStr=uint8  RndMeth=Round
  CAN1_LatAccCtrl : Outport
  wires:
  Data Type Conversion/1 -> CAN1_LatAccCtrl/1
  LatAccCtrl/1 -> Data Type Conversion/1

== system halout/HAL_OUT/CAN1/FD1_VMC1_0x17F/LateralCtrl ==
  LateralCtrl : Inport
  Data Type Conversion : DataTypeConversion  OutDataTypeStr=uint8  RndMeth=Round
  CAN1_LateralCtrl : Outport
  wires:
  Data Type Conversion/1 -> CAN1_LateralCtrl/1
  LateralCtrl/1 -> Data Type Conversion/1

== system halout/HAL_OUT/CAN1/FD1_VMC1_0x17F/LimitPCT ==
  LimitPCT : Inport
  Data Type Conversion : DataTypeConversion  OutDataTypeStr=uint8  RndMeth=Round
  CAN1_LimitPCT : Outport
  wires:
  Data Type Conversion/1 -> CAN1_LimitPCT/1
  LimitPCT/1 -> Data Type Conversion/1

== system halout/HAL_OUT/CAN1/FD1_VMC1_0x17F/MeterIndSpeedraw32 ==
  MeterIndSpeedraw32 : Inport
  Data Type Conversion : DataTypeConversion  OutDataTypeStr=uint8  RndMeth=Round
  CAN1_MeterIndSpeed_raw32 : Outport
  wires:
  Data Type Conversion/1 -> CAN1_MeterIndSpeed_raw32/1
  MeterIndSpeedraw32/1 -> Data Type Conversion/1

== system halout/HAL_OUT/CAN1/FD1_VMC1_0x17F/RearWhlSlipRatioCtrl ==
  RearWhlSlipRatioCtrl : Inport
  Data Type Conversion : DataTypeConversion  OutDataTypeStr=uint8  RndMeth=Round
  CAN1_RearWhlSlipRatioCtrl : Outport
  wires:
  Data Type Conversion/1 -> CAN1_RearWhlSlipRatioCtrl/1
  RearWhlSlipRatioCtrl/1 -> Data Type Conversion/1

== system halout/HAL_OUT/CAN1/FD1_VMC1_0x17F/SPD2ACCAct ==
  SPD2ACCAct : Inport
  Data Type Conversion : DataTypeConversion  OutDataTypeStr=uint8  RndMeth=Round
  CAN1_SPD2ACCAct : Outport
  wires:
  Data Type Conversion/1 -> CAN1_SPD2ACCAct/1
  SPD2ACCAct/1 -> Data Type Conversion/1

== system halout/HAL_OUT/CAN1/FD1_VMC1_0x17F/SafetyCtrl ==
  SafetyCtrl : Inport
  Data Type Conversion : DataTypeConversion  OutDataTypeStr=uint8  RndMeth=Round
  CAN1_SafetyCtrl : Outport
  wires:
  Data Type Conversion/1 -> CAN1_SafetyCtrl/1
  SafetyCtrl/1 -> Data Type Conversion/1

== system halout/HAL_OUT/CAN1/FD1_VMC1_0x17F/SingleWhlSlipRatioCtrl ==
  SingleWhlSlipRatioCtrl : Inport
  Data Type Conversion : DataTypeConversion  OutDataTypeStr=uint8  RndMeth=Round
  CAN1_SingleWhlSlipRatioCtrl : Outport
  wires:
  Data Type Conversion/1 -> CAN1_SingleWhlSlipRatioCtrl/1
  SingleWhlSlipRatioCtrl/1 -> Data Type Conversion/1

== system halout/HAL_OUT/CAN1/FD1_VMC1_0x17F/TimeGapCalcu ==
  TimeGapCalcu : Inport
  Data Type Conversion : DataTypeConversion  OutDataTypeStr=uint8  RndMeth=Round
  convert_out : FVT_lib/hal/convert_out  gain=0.1  offset=0
  CAN1_TimeGapCalcu : Outport
  wires:
  Data Type Conversion/1 -> CAN1_TimeGapCalcu/1
  convert_out/1 -> Data Type Conversion/1
  TimeGapCalcu/1 -> convert_out/1

== system halout/HAL_OUT/CAN1/FD1_VMC1_0x17F/VMCACCCtrlAvail ==
  VMCACCCtrlAvail : Inport
  Data Type Conversion : DataTypeConversion  OutDataTypeStr=uint8  RndMeth=Round
  CAN1_VMC_ACCCtrlAvail : Outport
  wires:
  Data Type Conversion/1 -> CAN1_VMC_ACCCtrlAvail/1
  VMCACCCtrlAvail/1 -> Data Type Conversion/1

== system halout/HAL_OUT/CAN1/FD1_VMC1_0x17F/VMCAEBCtrlAvail ==
  VMCAEBCtrlAvail : Inport
  Data Type Conversion : DataTypeConversion  OutDataTypeStr=uint8  RndMeth=Round
  CAN1_VMC_AEBCtrlAvail : Outport
  wires:
  Data Type Conversion/1 -> CAN1_VMC_AEBCtrlAvail/1
  VMCAEBCtrlAvail/1 -> Data Type Conversion/1

== system halout/HAL_OUT/CAN1/FD1_VMC1_0x17F/VMCCCCtrlAvail ==
  VMCCCCtrlAvail : Inport
  Data Type Conversion : DataTypeConversion  OutDataTypeStr=uint8  RndMeth=Round
  CAN1_VMC_CCCtrlAvail : Outport
  wires:
  Data Type Conversion/1 -> CAN1_VMC_CCCtrlAvail/1
  VMCCCCtrlAvail/1 -> Data Type Conversion/1

== system halout/HAL_OUT/CAN1/FD1_VMC1_0x17F/VMCMSACtrlAvail ==
  VMCMSACtrlAvail : Inport
  Data Type Conversion : DataTypeConversion  OutDataTypeStr=uint8  RndMeth=Round
  CAN1_VMC_MSACtrlAvail : Outport
  wires:
  Data Type Conversion/1 -> CAN1_VMC_MSACtrlAvail/1
  VMCMSACtrlAvail/1 -> Data Type Conversion/1

== system halout/HAL_OUT/CAN1/FD1_VMC1_0x17F/VMCVCUACCCtrlAvail ==
  VMCVCUACCCtrlAvail : Inport
  Data Type Conversion : DataTypeConversion  OutDataTypeStr=uint8  RndMeth=Round
  CAN1_VMC_VCU_ACC_CtrlAvail : Outport
  wires:
  Data Type Conversion/1 -> CAN1_VMC_VCU_ACC_CtrlAvail/1
  VMCVCUACCCtrlAvail/1 -> Data Type Conversion/1

== system halout/HAL_OUT/CAN1/FD1_VMC1_0x17F/VMCVCUAPSCtrlAvailflg ==
  VMCVCUAPSCtrlAvailflg : Inport
  Data Type Conversion : DataTypeConversion  OutDataTypeStr=uint8  RndMeth=Round
  CAN1_VMC_VCU_APSCtrlAvail_flg : Outport
  wires:
  Data Type Conversion/1 -> CAN1_VMC_VCU_APSCtrlAvail_flg/1
  VMCVCUAPSCtrlAvailflg/1 -> Data Type Conversion/1

== system halout/HAL_OUT/CAN1/FD1_VMC1_0x17F/VMCVCUAccPedalOverride ==
  VMCVCUAccPedalOverride : Inport
  Data Type Conversion : DataTypeConversion  OutDataTypeStr=uint8  RndMeth=Round
  CAN1_VMC_VCU_AccPedal_Override : Outport
  wires:
  Data Type Conversion/1 -> CAN1_VMC_VCU_AccPedal_Override/1
  VMCVCUAccPedalOverride/1 -> Data Type Conversion/1

== system halout/HAL_OUT/CAN1/FD1_VMC1_0x17F/VMCVCUCCCrlSta ==
  VMCVCUCCCrlSta : Inport
  Data Type Conversion : DataTypeConversion  OutDataTypeStr=uint8  RndMeth=Round
  CAN1_VMC_VCU_CC_Crl_Sta : Outport
  wires:
  Data Type Conversion/1 -> CAN1_VMC_VCU_CC_Crl_Sta/1
  VMCVCUCCCrlSta/1 -> Data Type Conversion/1

== system halout/HAL_OUT/CAN1/FD1_VMC1_0x17F/VMCVCUMSACrlSta ==
  VMCVCUMSACrlSta : Inport
  Data Type Conversion : DataTypeConversion  OutDataTypeStr=uint8  RndMeth=Round
  CAN1_VMC_VCU_MSA_Crl_Sta : Outport
  wires:
  Data Type Conversion/1 -> CAN1_VMC_VCU_MSA_Crl_Sta/1
  VMCVCUMSACrlSta/1 -> Data Type Conversion/1

== system halout/HAL_OUT/CAN1/FD1_VMC1_0x17F/VehicleSpeedkph ==
  VehicleSpeedkph : Inport
  Data Type Conversion : DataTypeConversion  OutDataTypeStr=uint16  RndMeth=Round
  convert_out : FVT_lib/hal/convert_out  gain=0.125  offset=0
  CAN1_VehicleSpeed_kph : Outport
  wires:
  Data Type Conversion/1 -> CAN1_VehicleSpeed_kph/1
  convert_out/1 -> Data Type Conversion/1
  VehicleSpeedkph/1 -> convert_out/1

== system halout/HAL_OUT/CAN1/FD1_VMC1_0x17F/VehicleSpeedmph ==
  VehicleSpeedmph : Inport
  Data Type Conversion : DataTypeConversion  OutDataTypeStr=uint16  RndMeth=Round
  convert_out : FVT_lib/hal/convert_out  gain=0.125  offset=0
  CAN1_VehicleSpeed_mph : Outport
  wires:
  Data Type Conversion/1 -> CAN1_VehicleSpeed_mph/1
  convert_out/1 -> Data Type Conversion/1
  VehicleSpeedmph/1 -> convert_out/1

== system halout/HAL_OUT/CAN1/FD1_VMC2_0x77/FDCVMCRWSActvSta ==
  FDCVMCRWSActvSta : Inport
  Data Type Conversion : DataTypeConversion  OutDataTypeStr=uint8  RndMeth=Round
  CAN1_FDC_VMC_RWS_Actv_Sta : Outport
  wires:
  Data Type Conversion/1 -> CAN1_FDC_VMC_RWS_Actv_Sta/1
  FDCVMCRWSActvSta/1 -> Data Type Conversion/1

== system halout/HAL_OUT/CAN1/FD1_VMC2_0x77/FDCVMCRWSDfctvSta ==
  FDCVMCRWSDfctvSta : Inport
  Data Type Conversion : DataTypeConversion  OutDataTypeStr=uint8  RndMeth=Round
  CAN1_FDC_VMC_RWS_Dfctv_Sta : Outport
  wires:
  Data Type Conversion/1 -> CAN1_FDC_VMC_RWS_Dfctv_Sta/1
  FDCVMCRWSDfctvSta/1 -> Data Type Conversion/1

== system halout/HAL_OUT/CAN1/FD1_VMC2_0x77/FDCVMCRWSPositionReqCmd ==
  FDCVMCRWSPositionReqCmd : Inport
  Data Type Conversion : DataTypeConversion  OutDataTypeStr=uint16  RndMeth=Round
  convert_out : FVT_lib/hal/convert_out  gain=0.01  offset=-327.67
  CAN1_FDC_VMC_RWS_PositionReq_Cmd : Outport
  wires:
  Data Type Conversion/1 -> CAN1_FDC_VMC_RWS_PositionReq_Cmd/1
  convert_out/1 -> Data Type Conversion/1
  FDCVMCRWSPositionReqCmd/1 -> convert_out/1

== system halout/HAL_OUT/CAN1/FD1_VMC2_0x77/FDCVMCSteerFaultReqCmd ==
  FDCVMCSteerFaultReqCmd : Inport
  Data Type Conversion : DataTypeConversion  OutDataTypeStr=uint8  RndMeth=Round
  CAN1_FDC_VMC_SteerFaultReq_Cmd : Outport
  wires:
  Data Type Conversion/1 -> CAN1_FDC_VMC_SteerFaultReq_Cmd/1
  FDCVMCSteerFaultReqCmd/1 -> Data Type Conversion/1

== system halout/HAL_OUT/CAN1/VMC_FCM1_0x172/Byte_0 ==
  VMC_FCM1_Checksum : Inport
  BitwiseOR : simulink/Logic and Bit Operations/Bitwise Operator  logicop=OR  UseBitMask=off  BitMask=bin2dec('11011001')  BitMaskRealWorld=Stored Integer
  SignalPack : FVT_lib/hal/SignalPack  RightShiftCnt=0  BitMask=2^8-1  LeftShiftCnt=0
  UnitConverter : DataTypeConversion  OutDataTypeStr=uint8  RndMeth=Round
  UnitConverter1 : DataTypeConversion  OutDataTypeStr=uint8  RndMeth=Round
  Byte_0 : Outport
  wires:
  BitwiseOR/1 -> Byte_0/1
  UnitConverter/1 -> BitwiseOR/1
  SignalPack/1 -> UnitConverter/1
  UnitConverter1/1 -> SignalPack/1
  VMC_FCM1_Checksum/1 -> UnitConverter1/1

== system halout/HAL_OUT/CAN1/VMC_FCM1_0x172/Byte_1 ==
  VMC_FCM1_LifeCount : Inport
  BitwiseOR : simulink/Logic and Bit Operations/Bitwise Operator  logicop=OR  UseBitMask=off  BitMask=bin2dec('11011001')  BitMaskRealWorld=Stored Integer
  SignalPack : FVT_lib/hal/SignalPack  RightShiftCnt=0  BitMask=2^4-1  LeftShiftCnt=0
  UnitConverter : DataTypeConversion  OutDataTypeStr=uint8  RndMeth=Round
  UnitConverter1 : DataTypeConversion  OutDataTypeStr=uint8  RndMeth=Round
  Byte_1 : Outport
  wires:
  BitwiseOR/1 -> Byte_1/1
  UnitConverter/1 -> BitwiseOR/1
  SignalPack/1 -> UnitConverter/1
  UnitConverter1/1 -> SignalPack/1
  VMC_FCM1_LifeCount/1 -> UnitConverter1/1

== system halout/HAL_OUT/CAN1/VMC_FCM1_0x172/Byte_10 ==
  VMC_ACC_ComfortBandLower : Inport
  BitwiseOR : simulink/Logic and Bit Operations/Bitwise Operator  logicop=OR  UseBitMask=off  BitMask=bin2dec('11011001')  BitMaskRealWorld=Stored Integer
  SignalPack : FVT_lib/hal/SignalPack  RightShiftCnt=0  BitMask=2^8-1  LeftShiftCnt=0
  UnitConverter : DataTypeConversion  OutDataTypeStr=uint8  RndMeth=Round
  UnitConverter1 : DataTypeConversion  OutDataTypeStr=uint16  RndMeth=Round
  convert_out : FVT_lib/hal/convert_out  gain=0.05  offset=-15
  Byte_10 : Outport
  wires:
  BitwiseOR/1 -> Byte_10/1
  UnitConverter/1 -> BitwiseOR/1
  SignalPack/1 -> UnitConverter/1
  UnitConverter1/1 -> SignalPack/1
  convert_out/1 -> UnitConverter1/1
  VMC_ACC_ComfortBandLower/1 -> convert_out/1

== system halout/HAL_OUT/CAN1/VMC_FCM1_0x172/Byte_11 ==
  FDC_VMC_DrInpTqBstAct : Inport
  FDC_VMC_MaxAngCtrlOutTqLim : Inport  Port=2
  VMC_ADAS_ACC_Sta : Inport  Port=3
  VMC_ADAS_AEB_Sta : Inport  Port=4
  BitwiseOR : simulink/Logic and Bit Operations/Bitwise Operator  logicop=OR  UseBitMask=off  NumInputPorts=4  BitMask=bin2dec('11011001')  BitMaskRealWorld=Stored Integer
  SignalPack : FVT_lib/hal/SignalPack  RightShiftCnt=0  BitMask=2^1-1  LeftShiftCnt=1
  SignalPack1 : FVT_lib/hal/SignalPack  RightShiftCnt=8  BitMask=2^1-1  LeftShiftCnt=0
  SignalPack2 : FVT_lib/hal/SignalPack  RightShiftCnt=0  BitMask=2^3-1  LeftShiftCnt=5
  SignalPack3 : FVT_lib/hal/SignalPack  RightShiftCnt=0  BitMask=2^3-1  LeftShiftCnt=2
  UnitConverter{,1..2,4..7} (7 alike) : DataTypeConversion  OutDataTypeStr=uint8  RndMeth=Round
  UnitConverter3 : DataTypeConversion  OutDataTypeStr=uint16  RndMeth=Round
  convert_out : FVT_lib/hal/convert_out  gain=0.1  offset=0
  Byte_11 : Outport
  wires:
  BitwiseOR/1 -> Byte_11/1
  UnitConverter/1 -> BitwiseOR/1
  SignalPack/1 -> UnitConverter/1
  UnitConverter1/1 -> SignalPack/1
  FDC_VMC_DrInpTqBstAct/1 -> UnitConverter1/1
  UnitConverter2/1 -> BitwiseOR/2
  SignalPack1/1 -> UnitConverter2/1
  UnitConverter3/1 -> SignalPack1/1
  convert_out/1 -> UnitConverter3/1
  FDC_VMC_MaxAngCtrlOutTqLim/1 -> convert_out/1
  UnitConverter4/1 -> BitwiseOR/3
  SignalPack2/1 -> UnitConverter4/1
  UnitConverter5/1 -> SignalPack2/1
  VMC_ADAS_ACC_Sta/1 -> UnitConverter5/1
  UnitConverter6/1 -> BitwiseOR/4
  SignalPack3/1 -> UnitConverter6/1
  UnitConverter7/1 -> SignalPack3/1
  VMC_ADAS_AEB_Sta/1 -> UnitConverter7/1

== system halout/HAL_OUT/CAN1/VMC_FCM1_0x172/Byte_12 ==
  FDC_VMC_MaxAngCtrlOutTqLim : Inport
  BitwiseOR : simulink/Logic and Bit Operations/Bitwise Operator  logicop=OR  UseBitMask=off  BitMask=bin2dec('11011001')  BitMaskRealWorld=Stored Integer
  SignalPack : FVT_lib/hal/SignalPack  RightShiftCnt=0  BitMask=2^8-1  LeftShiftCnt=0
  UnitConverter : DataTypeConversion  OutDataTypeStr=uint8  RndMeth=Round
  UnitConverter1 : DataTypeConversion  OutDataTypeStr=uint16  RndMeth=Round
  convert_out : FVT_lib/hal/convert_out  gain=0.1  offset=0
  Byte_12 : Outport
  wires:
  BitwiseOR/1 -> Byte_12/1
  UnitConverter/1 -> BitwiseOR/1
  SignalPack/1 -> UnitConverter/1
  UnitConverter1/1 -> SignalPack/1
  convert_out/1 -> UnitConverter1/1
  FDC_VMC_MaxAngCtrlOutTqLim/1 -> convert_out/1
